simulink model "Ball_Estimation_27_12"  (Simulink 8.0)
settings: Solver=ode4  StartTime=0.0  StopTime=inf  FixedStep=sample_time  RelTol=1e-3
InitFcn:
  | sample_time=0.005;%0.004;%0.0025;%0.02;
  | sample_time_Vicon = 0.005;
  | DeltaT = 0.02;
  | g = 9.81;
  | H0 = g%0.3165;
  | 
  | Q6_mass = 0.7;
  | 
  | Q6_Omega_r = 1.6; %for horizon ref
  | Q6_Zeta_r = 0.5; %for horizon ref
  | Q6_Omega_r_h = 2;%for vertical ref
  | Q6_Zeta_r_h = 1; %for vertical ref
  | 
  | 
  | Q6_Omega = 1.5; %for horizon control
  | Q6_Zeta = 0.5; %for horizon control
  | Q6_Omega_h= 2; %for vertical control
  | Q6_Zeta_h = 0.7; %for vertical control
  | 
  | 
  | Q6_acc_max = 5;%horizontal max acc
  | Q6_acc_max_h = 3;%horizontal max acc
  | 
  | omega_circle = 72*pi/180;
  | omega_h = 0.1;%Ascending speed
  | PI = pi;
  | Circle_R = 2.5;
  | MAX_Height = -2;
undefined symbols (not defined in the file or in its folder): DiscIntNeverNeededParam, PosRefSystem, X330_Control
libraries: simulink x2, dspadpt3 x2
(part 2 of 2)

== stateflow chart Estimation/Trajectory Logic1/UAV SF ==
  state Airborne
    state Standby
    state Calculation
      en:
      [Pe,T]=TrajEst(x,y,z,zd,Peo[0],Peo[1],To);
      x[0] = x[1];x[1] = x[2];x[2] = x[3];x[3] = x[4];
      y[0] = y[1];y[1] = y[2];y[2] = y[3];y[3] = y[4];
      z[0] = z[1];z[1] = z[2];z[2] = z[3];z[3] = z[4];
    state Getdata
      en:
      x[i] = Sc_Pos[0];
      y[i] = Sc_Pos[1];
      z[i] = Sc_Pos[2];
    state Output1
      en:
      ImpactPoint = Pe;
      DesiredTime = T;
    state daq
      en:
      i=i+1;
    state Output2
      en:
      ImpactPoint[0] = 0;
      ImpactPoint[1] = 0;
      ImpactPoint[2] = zd;
      DesiredTime = 0;
    Output1 -> (junction 19) : {i=i-2;}
    (default) -> Standby : {i=-1;Peo=0;To=0;}
    (junction 20) -> (junction 19) [order 1] : [(Sc_Vel[2]<-1)&(Sc_Vel[2]>-6)]
    Standby -> (junction 20) : [(abs(Sc_Pos[0]) <= 4.5)&(abs(Sc_Pos[1])<=4.5)&(abs(Sc_Pos[2])<=4)]
    (junction 19) -> daq [order 2]
    (junction 20) -> Output2 [order 2]
    Output2 -> Standby
    (junction 19) -> Output2 [order 1] : [(Sc_Pos[2] >= -0.8)&(Sc_Vel[2]>0)]
    Getdata -> daq
    daq -> Getdata [order 1] : [i==0]
    (junction 21) -> Getdata [order 1] : [(x[i-1]~=Sc_Pos[0])||(y[i-1]~=Sc_Pos[1])||(z[i-1]~=Sc_Pos[2])]
    daq -> (junction 21) [order 3] : [(i>0)&(i<5)]
    (junction 21) -> daq [order 2] : {i=i-1;}
    daq -> Calculation [order 2] : [i==5]
    Calculation -> Output1 : {Peo=Pe;To=T;}
  data: xi function_input double size=5; yi function_input double size=5; zi function_input double size=5; Pe function_output double size=3; T function_output double size=1; zd function_input double size=1; t0 constant double size=5 =[0 0.005 0.01 0.015 0.02]; xo function_input double; yo function_input double; To function_input double; ImpactPoint output double size=3; DesiredTime output double size=1; Sc_Pos input double size=3; Sc_Vel input double size=3; DeltaT parameter double size=1; T local double size=1; zd local double size=1 =-0.8; Pe local double size=3; i local double; x local double size=5 =[0 0 0 0 0 ]; y local double size=5 =[0 0 0 0 0 ]; z local double size=5 =[0 0 0 0 0 ]; Peo local double size=3; To local double size=1; Pe1 local double size=3; T1 local double size=1
  function [Pe,T]=TrajEst(xi,yi,zi,zd,xo,yo,To):
    | function [Pe,T]=TrajEst(xi,yi,zi,zd,xo,yo,To)
    | 
    | p=polyfit(t0,zi,2)';
    | a=p(1);
    | b=p(2);
    | c=p(3);
    | 
    | 
    | xe=0;
    | ye=0;
    | T=0;
    | if((To>0)&&(To<1.2))
    |     xe = xo;
    |     ye = yo;
    |     T = To;
    | end;
    | if(a > 3)
    |     if(b^2 - 4*a*(c-zd) >= 0)
    |         T=(-b+sqrt(b^2 - 4*a*(c-zd)))/(2*a);
    |         xe=polyval(polyfit(t0,xi,1),T);
    |         ye=polyval(polyfit(t0,yi,1),T);
    |     end;
    | 
    |     if((To>0)&&(To<1.2))
    |         if((T>1.2)||(abs(xe)>4)||(abs(ye)>4))
    |             T = To;
    |             xe = xo;
    |             ye = yo;
    |         else
    |             T = 0.7*T + 0.3*(To-0.005);
    |             xe = 0.7*xo + 0.3*xe;
    |             ye = 0.7*yo + 0.3*ye;
    |         end
    |     else
    |        if((T>1.2)||(xe<-1.5)||(xe>2.5)||(ye<-2.5)||(ye>2.5)) 
    |            xe=0;
    |            ye=0;
    |            T=0;
    |        end;
    |     end;
    | end
    | 
    | Pe=[xe ye zd]';

== matlab function UAV 1/Yaw Controller/MATLAB Function ==
  data: u input double; y output double
function y = fcn(u)
%#codegen
y = u;
if y > pi    
    y = y - 2*pi;
elseif y < -pi
        y = y + 2*pi;
end

== stateflow chart UAV 1/Trajectory Logic/UAV SF1 ==
  state Landing
    state Decsending
      en:PosDesired = Pos;
      du:PosDesired[2] = (0 - PosDesired[2])*1*DeltaT + PosDesired[2] ;
    state CutThrottle
      du:HoverThrottle = (0.01 - HoverThrottle)*2*DeltaT + HoverThrottle ;
    (default) -> Decsending
    Decsending -> CutThrottle : [Pos[2] > -0.15]
  state Airborne1
    state TakeOff
      du:HoverThrottle = (H0 - HoverThrottle)*2*DeltaT + HoverThrottle ;
    state Trajectory
      en:
      PosDesired[0] = 2.5*ImpactPoint[0]-1.5*Pos[0];
      PosDesired[1] = 2.5*ImpactPoint[1]-1.5*Pos[0];
      Takeoff=1;
    state Hover
      en:
      PosDesired[0] = 0;
      PosDesired[1] = 0;
      PosDesired[2] = -0.6;
      Takeoff=1;
    (default) -> TakeOff : {PosDesired = Pos;  PosDesired[2] = -1;Takeoff=0;}
    (junction 81) -> Trajectory [order 1] : [Pos[2]<-0.4]
    (junction 81) -> Hover [order 2]
    (junction 82) -> (junction 81) [order 2]
    TakeOff -> Hover : [RC[5]>0.5]
        | {PosDesired = Pos;try=1;}
    Trajectory -> (junction 83)
    (junction 82) -> Hover [order 1] : [RC[5]<-0.5]
    (junction 83) -> (junction 82) [order 1] : [(ImpactPoint[0]<xmax)&(ImpactPoint[0]>xmin)&(ImpactPoint[1]<ymax)&(ImpactPoint[1]>ymin)]
    (junction 83) -> Hover [order 2]
    Hover -> (junction 83) [order 1] : [(ImpactPoint[0] ~= 0)&(ImpactPoint[1]~= 0)]
    Hover -> Hover [order 2]
  Landing -> Airborne1 : [RC[6] > 0.5]
  Airborne1 -> Landing : [RC[6] < -0.5]
  (default) -> Landing : {HoverThrottle=0.01;}
  data: PosDesired output double size=4; HoverThrottle output double size=1; RC input double size=8; Pos input double size=4; ImpactPoint input double size=3; DeltaT parameter double size=1; H0 parameter double size=1; zmax constant double size=1 =-2.5; Takeoff output double size=1; DesiredTime input double size=1; xmax constant double size=1 =2; xmin constant double size=1 =-1; ymax constant double size=1 =1; ymin constant double size=1 =-1; try local double
